simulink model "modelo_real"  (R2018b)
settings: Solver=ode4  StartTime=0.0  StopTime=t_f  FixedStep=fst  RelTol=1e-3  EnableMultiTasking=on
values from neighbouring files (symbols this model uses):
  b = 0.1210    (= 0.121)    [Script_principal.m]
  c_d = r_d/(2*b)    (= 0.120661157025)    [Script_principal.m]
  c_e = r_e/(2*b)    (= 0.121074380165)    [Script_principal.m]
  delayD = 0.1/fst    (= 100)    [Script_principal.m]
  delayE = 0.1/fst    (= 100)    [Script_principal.m]
  fD_v = var_fD*0.0069    (= 0.0069)    [Script_principal.m]
  fE_v = var_fE*0.0053    (= 0.0053)    [Script_principal.m]
  filter_order = 2    [Script_principal.m]
  freq_pos = 200    [Script_principal.m]
  freq_vel = 200    [Script_principal.m]
  I_v = var_I*0.0903    (= 0.0903)    [Script_principal.m]
  Ir_v = var_Ir*0.00094    (= 0.00094)    [Script_principal.m]
  k0 = 25    [Script_principal.m]
  k1 = 25    [Script_principal.m]
  k_enc = 2*pi/fpr    (= 0.157079632679)    [Script_principal.m]
  KaD_v = var_KaD*0.4713    (= 0.4713)    [Script_principal.m]
  KaE_v = var_KaE*0.5046    (= 0.5046)    [Script_principal.m]
  KtD_v = var_KtD*KaD    (= 0.4713)    [Script_principal.m]
  KtE_v = var_KtE*KaE    (= 0.5046)    [Script_principal.m]
  L = 0.10    (= 0.1)    [Script_principal.m]
  m_v = var_m*1.932    (= 1.932)    [Script_principal.m]
  r_d = 0.0292    [Script_principal.m]
  r_e = 0.0293    [Script_principal.m]
  RaD_v = var_RaD*8.4507    (= 8.4507)    [Script_principal.m]
  RaE_v = var_RaE*7.7177    (= 7.7177)    [Script_principal.m]
  svzD = 0    [Script_principal.m]
  svzE = 0    [Script_principal.m]
  T = 3    [Script_principal.m]
  VaD_max = 14    [Script_principal.m]
  VaD_min = 2    [Script_principal.m]
  VaE_max = 14    [Script_principal.m]
  VaE_min = 2    [Script_principal.m]
  x0_1 = -L    (= -0.1)    [Script_principal.m]
  x0_2 = 0    [Script_principal.m]
  x0_3 = 0    [Script_principal.m]
  x0_4 = 0    [Script_principal.m]
  x0_5 = 0    [Script_principal.m]
  x0_6 = 0    [Script_principal.m]
undefined symbols (not defined in the file or in its folder): a, dur_c, t_f, t_i, t_i_1, t_i_2, t_i_3, t_i_c, time_c, v, w, wx, wy
libraries: simulink x39, embdlinuxlib x7, dspmtrx3 x6, cstblocks x4, raspberrypilib x1
(part 2 of 2)

== matlab function modelo_real/Equação Linearizante/Equação Linearizante ==
  data: cte input; u input; x input; micro output
function micro = fcn(cte, u, x)
%#codegen
% Parametros de simulação--------------------------------------------------
% micro = µ;
% eta = η;

b   = cte(1,1);
c_d = cte(1,2);
c_e = cte(1,3);
L   = cte(1,4);

%--------------------------------------------------------------------------
thetaD_d = x(5,1);
thetaE_d = x(6,1);
phi      = c_d*x(3,1)-c_e*x(4,1);

%--------------------------------------------------------------------------
LgLfh = [c_d*b*cos(phi)-c_d*L*sin(phi) c_e*b*cos(phi)+c_e*L*sin(phi);
         c_d*b*sin(phi)+c_d*L*cos(phi) c_e*b*sin(phi)-c_e*L*cos(phi)];
     
LfLfh = [-(c_d^2*b*sin(phi)+c_d^2*L*cos(phi))*thetaD_d^2 + (c_e^2*b*sin(phi)-c_e^2*L*cos(phi))*thetaE_d^2 + 2*c_d*c_e*L*cos(phi)*thetaD_d*thetaE_d;
          (c_d^2*b*cos(phi)-c_d^2*L*sin(phi))*thetaD_d^2 - (c_e^2*b*cos(phi)+c_e^2*L*sin(phi))*thetaE_d^2 + 2*c_d*c_e*L*sin(phi)*thetaD_d*thetaE_d];
   
%--------------------------------------------------------------------------
micro = LgLfh^-1*(u-LfLfh);

== matlab function modelo_real/Saída/Saídas ==
  data: xr output; yr output; xr_d output; yr_d output; cte input; x input
function [xr, yr, xr_d, yr_d] = fcn(cte, x)
%#codegen
% Parametros de simulação--------------------------------------------------

b   = cte(1,1);
c_d = cte(1,2);
c_e = cte(1,3);
L   = cte(1,4);

%--------------------------------------------------------------------------
xo       = x(1,1);
yo       = x(2,1);
thetaD_d = x(5,1);
thetaE_d = x(6,1);
phi      = c_d*x(3,1)-c_e*x(4,1);

%--------------------------------------------------------------------------
Lfh = [c_d*b*cos(phi)*thetaD_d+c_e*b*cos(phi)*thetaE_d-c_d*L*sin(phi)*thetaD_d+c_e*L*sin(phi)*thetaE_d;
       c_d*b*sin(phi)*thetaD_d+c_e*b*sin(phi)*thetaE_d+c_d*L*cos(phi)*thetaD_d-c_e*L*cos(phi)*thetaE_d];

xr_d = Lfh(1,1);
yr_d = Lfh(2,1);

xr = xo + L*cos(phi);
yr = yo + L*sin(phi);

== matlab function modelo_real/Cancelamento da dinâmica/Transformação da Entrada ==
  data: cte input; micro input; x input; tauD output; tauE output
function [tauD, tauE] = fcn(cte, micro, x)
%#codegen
% Parametros de simulação--------------------------------------------------
% eta = η;

b   = cte(1,1);
r_d = cte(1,2);
r_e = cte(1,3);
c_d = cte(1,4);
c_e = cte(1,5);
Ir  = cte(1,6);
m   = cte(1,7);
I   = cte(1,8);

%--------------------------------------------------------------------------
thetaD_d = x(5,1);
thetaE_d = x(6,1);
phi      = c_d*x(3,1)-c_e*x(4,1);

%--------------------------------------------------------------------------
S = [ c_d*b*cos(phi) , c_e*b*cos(phi) ;
      c_d*b*sin(phi) , c_e*b*sin(phi) ;
            1        ,       0        ;
            0        ,       1        ];
               
S_d = [ -(r_d^2/4*b)*sin(phi)*thetaD_d + (r_d*r_e/4*b)*sin(phi)*thetaE_d , -(r_d*r_e/4*b)*sin(phi)*thetaD_d + (r_e^2/4*b)*sin(phi)*thetaE_d;
         (r_d^2/4*b)*cos(phi)*thetaD_d - (r_d*r_e/4*b)*cos(phi)*thetaE_d ,  (r_d*r_e/4*b)*cos(phi)*thetaD_d - (r_e^2/4*b)*cos(phi)*thetaE_d;
                                       0                                 ,                                  0                              ;
                                       0                                 ,                                  0                              ];
                        
M = [ m , 0 ,       0    ,       0    ;
      0 , m ,       0    ,       0    ;
      0 , 0 , Ir+I*c_d^2 ,   -I*c_e^2 ;
      0 , 0 ,   -I*c_d^2 , Ir+I*c_e^2 ];
            
eta = [thetaD_d;
       thetaE_d];
   
% Cálculo de tau-----------------------------------------------------------

tau  = (S'*M*S_d*eta) + S'*M*S*micro;
tauD = tau(1,1);
tauE = tau(2,1);
